simulink model "presse_example"  (R2020b)
settings: Solver=FixedStepAuto  StartTime=0.0  StopTime=90  FixedStep=0.01  RelTol=1e-3
InitFcn:
  | config_presse
values from neighbouring files (symbols this model uses):
  G_s = 0.15    [config_presse.m]
  t_09 = 15    [config_presse.m]
  T_max = 90    [config_presse.m]
  T_min = -40    [config_presse.m]
settings Model: EnablePacing=on  Creator=mateu  LastModifiedBy=mateu

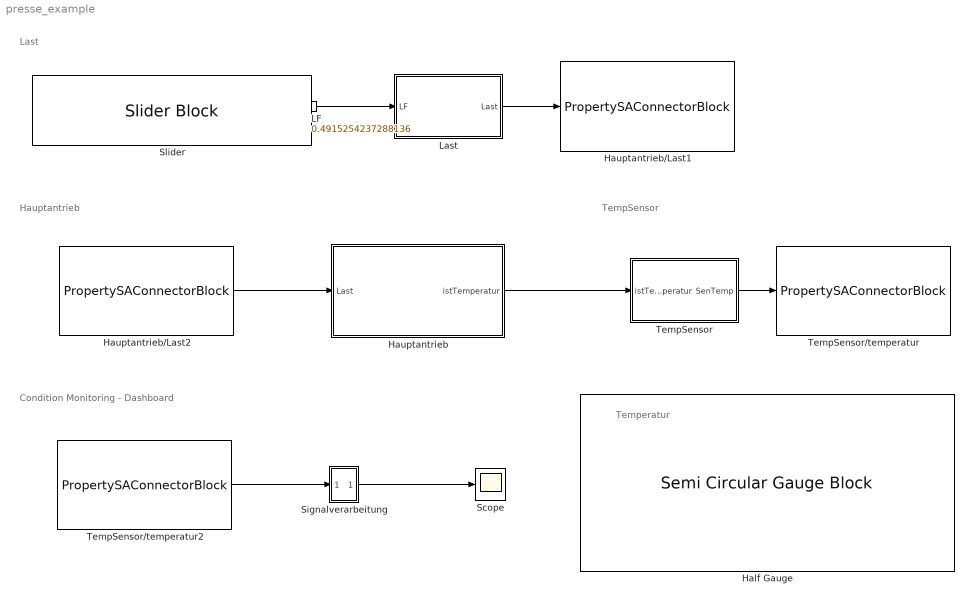
== system presse_example ==
  note: Temperatur
  note: TempSensor
  note: Last
  note: Hauptantrieb
  note: Condition Monitoring - Dashboard
  Half Gauge : SemiCircularGaugeBlock  LabelPosition=Hide  ScaleMin=-10
  Hauptantrieb : Subsystem
  Hauptantrieb/Last1 : S-Function  FunctionName=PropertySAConnectorBlock  Parameters=sr, regUrlStr, aasId, smId, seId  SFunctionDeploymentMode=off  EnableBusSupport=off  mask{sr=0.5, regUrlStr=http://localhost:8082/registry/api/v1/registry, aasId=https://example.com/ids/aas/6001_2130_8022_6165, smId=Hauptantrieb, seId=last}
      mask prompts: sr "Sample Rate"; regUrlStr "Registry URL"; aasId "AAS Id"; smId "Submodel IdShort"; seId "Property IdShort"
      mask Display:
      | sr = get_param(gcb,'sr')
      | aas = replace(get_param(gcb,'aasId'),"_","\_");
      | sm = replace(get_param(gcb,'smId'),"_","\_");
      | se = replace(get_param(gcb,'seId'),"_","\_");
      | 
      | pos = get_param(gcb, 'Position');
      | w = pos(3) - pos(1);
      | h = pos(4) - pos(2);
      | 
      | full = sm  + "/" + se
      | text(5,20, "{\bf\fontsize{7}"+aas+"}", 'texmode','on')
      | text(5,10, "{\bf\fontsize{6}"+full+"}", 'texmode','on')
      | image('basyx.png', [w-15,h-20,10,15]);
      | port_label('output', 1,"{\bf\fontsize{6}sr="+sr+"s}", 'texmode','on')
  Hauptantrieb/Last2 : S-Function  FunctionName=PropertySAConnectorBlock  Parameters=sr, regUrlStr, aasId, smId, seId  SFunctionDeploymentMode=off  EnableBusSupport=off  mask{sr=0.5, regUrlStr=http://localhost:8082/registry/api/v1/registry, aasId=https://example.com/ids/aas/6001_2130_8022_6165, smId=Hauptantrieb, seId=last}
      mask prompts: sr "Sample Rate"; regUrlStr "Registry URL"; aasId "AAS Id"; smId "Submodel IdShort"; seId "Property IdShort"
      mask Display:
      | sr = get_param(gcb,'sr')
      | aas = replace(get_param(gcb,'aasId'),"_","\_");
      | sm = replace(get_param(gcb,'smId'),"_","\_");
      | se = replace(get_param(gcb,'seId'),"_","\_");
      | 
      | pos = get_param(gcb, 'Position');
      | w = pos(3) - pos(1);
      | h = pos(4) - pos(2);
      | 
      | full = sm  + "/" + se
      | text(5,20, "{\bf\fontsize{7}"+aas+"}", 'texmode','on')
      | text(5,10, "{\bf\fontsize{6}"+full+"}", 'texmode','on')
      | image('basyx.png', [w-15,h-20,10,15]);
      | port_label('output', 1,"{\bf\fontsize{6}sr="+sr+"s}", 'texmode','on')
  LF : Constant  Value=0.4915254237288136
  Last : Subsystem
  Scope : Scope
  Signalverarbeitung : Subsystem
  Slider : SliderBlock  ScaleMax=1  TickInterval=0.1
  TempSensor : Subsystem
  TempSensor/temperatur : S-Function  FunctionName=PropertySAConnectorBlock  Parameters=sr, regUrlStr, aasId, smId, seId  SFunctionDeploymentMode=off  EnableBusSupport=off  mask{sr=0.1, regUrlStr=http://localhost:8082/registry/api/v1/registry, aasId=https://example.com/ids/aas/6001_2130_8022_6165, smId=TempSensor, seId=temperatur}
      mask prompts: sr "Sample Rate"; regUrlStr "Registry URL"; aasId "AAS Id"; smId "Submodel IdShort"; seId "Property IdShort"
      mask Display:
      | sr = get_param(gcb,'sr')
      | aas = replace(get_param(gcb,'aasId'),"_","\_");
      | sm = replace(get_param(gcb,'smId'),"_","\_");
      | se = replace(get_param(gcb,'seId'),"_","\_");
      | 
      | pos = get_param(gcb, 'Position');
      | w = pos(3) - pos(1);
      | h = pos(4) - pos(2);
      | 
      | full = sm  + "/" + se
      | text(5,20, "{\bf\fontsize{7}"+aas+"}", 'texmode','on')
      | text(5,10, "{\bf\fontsize{6}"+full+"}", 'texmode','on')
      | image('basyx.png', [w-15,h-20,10,15]);
      | port_label('output', 1,"{\bf\fontsize{6}sr="+sr+"s}", 'texmode','on')
  TempSensor/temperatur2 : S-Function  FunctionName=PropertySAConnectorBlock  Parameters=sr, regUrlStr, aasId, smId, seId  SFunctionDeploymentMode=off  EnableBusSupport=off  mask{sr=0.1, regUrlStr=http://localhost:8082/registry/api/v1/registry, aasId=https://example.com/ids/aas/6001_2130_8022_6165, smId=TempSensor, seId=temperatur}
      mask prompts: sr "Sample Rate"; regUrlStr "Registry URL"; aasId "AAS Id"; smId "Submodel IdShort"; seId "Property IdShort"
      mask Display:
      | sr = get_param(gcb,'sr')
      | aas = replace(get_param(gcb,'aasId'),"_","\_");
      | sm = replace(get_param(gcb,'smId'),"_","\_");
      | se = replace(get_param(gcb,'seId'),"_","\_");
      | 
      | pos = get_param(gcb, 'Position');
      | w = pos(3) - pos(1);
      | h = pos(4) - pos(2);
      | 
      | full = sm  + "/" + se
      | text(5,20, "{\bf\fontsize{7}"+aas+"}", 'texmode','on')
      | text(5,10, "{\bf\fontsize{6}"+full+"}", 'texmode','on')
      | image('basyx.png', [w-15,h-20,10,15]);
      | port_label('output', 1,"{\bf\fontsize{6}sr="+sr+"s}", 'texmode','on')
  wires:
  Hauptantrieb/Last2/1 -> Hauptantrieb/1(Last)
  TempSensor/temperatur2/1 -> Signalverarbeitung/1(In1)
  Signalverarbeitung/1(Out1) -> Scope/1
  LF/1 -> Last/1(LF)
  Hauptantrieb/1(istTemperatur) -> TempSensor/1(istTemperatur)
  TempSensor/1(SenTemp) -> TempSensor/temperatur/1
  Last/1(Last) -> Hauptantrieb/Last1/1

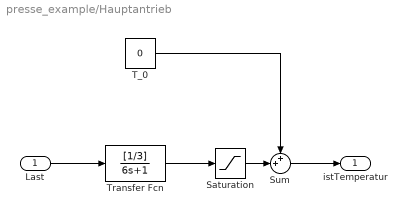
== system presse_example/Hauptantrieb ==
  Last : Inport
  Saturation : Saturate  UpperLimit=150  LowerLimit=0
  Sum : Sum  Inputs=++|
  T_0 : Constant  Value=0
  Transfer Fcn : TransferFcn  Numerator=[1/3]  Denominator=[6 1]
  istTemperatur : Outport
  wires:
  Last/1 -> Transfer Fcn/1
  T_0/1 -> Sum/1
  Sum/1 -> istTemperatur/1
  Transfer Fcn/1 -> Saturation/1
  Saturation/1 -> Sum/2

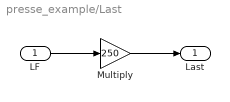
== system presse_example/Last ==
  LF : Inport
  Multiply : Gain  Gain=250
  Last : Outport
  wires:
  Multiply/1 -> Last/1
  LF/1 -> Multiply/1

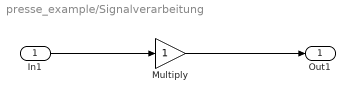
== system presse_example/Signalverarbeitung ==
  In1 : Inport
  Multiply : Gain
  Out1 : Outport
  wires:
  Multiply/1 -> Out1/1
  In1/1 -> Multiply/1

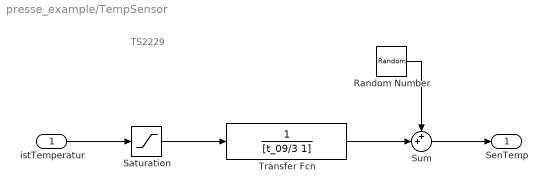
== system presse_example/TempSensor ==
  note: TS2229
  istTemperatur : Inport
  Random Number : RandomNumber  Variance=G_s/32  Seed=202021
  Saturation : Saturate  UpperLimit=T_max  LowerLimit=T_min
  Sum : Sum  Inputs=++|
  Transfer Fcn : TransferFcn  Denominator=[t_09/3 1]
  SenTemp : Outport
  wires:
  Transfer Fcn/1 -> Sum/2
  Saturation/1 -> Transfer Fcn/1
  Sum/1 -> SenTemp/1
  istTemperatur/1 -> Saturation/1
  Random Number/1 -> Sum/1
